simulink model "Karnop"  (R2015b)
settings: Solver=VariableStepAuto  StartTime=0.0  StopTime=10.0  RelTol=1e-3
values from neighbouring files (symbols this model uses):
  d_v = 10    [ex1.m]    (also in ex2.m = 1; ex3.m; ex4.m = 1; exall.m = 1)
  F_c = 0.001    [ex1.m]    (also in ex2.m; ex3.m; ex4.m; exall.m)
  motor_L = motor_pars    [ex1.m]    (also in ex2.m; ex3.m; ex4.m)
libraries: simulink x1
settings Model: Creator=Andreas  LastModifiedBy=Andreas

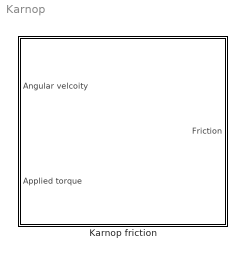
== system Karnop ==
  Karnop friction : Subsystem

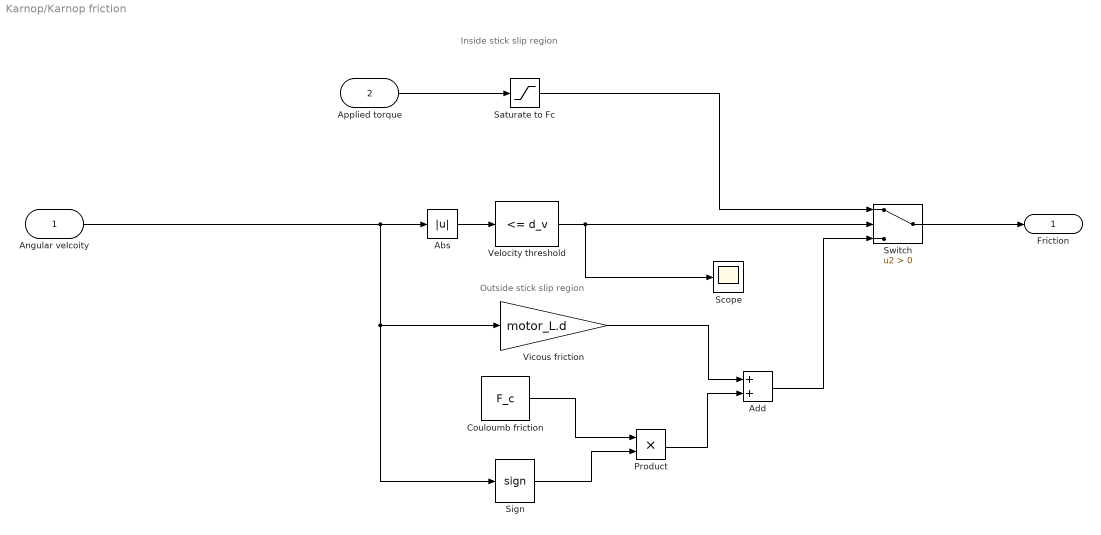
== system Karnop/Karnop friction ==
  note: Outside stick slip region
  note: Inside stick slip region
  Angular velcoity : Inport
  "Applied torque " : Inport  Port=2
  Abs : Abs
  Add : Sum
  Couloumb friction : Constant  Value=F_c
  Product : Product
  Saturate to Fc : Saturate  UpperLimit=F_c  LowerLimit=-F_c
  Scope : Scope
  Sign : Signum
  Switch : Switch  Criteria=u2 > Threshold
  "Velocity threshold " : simulink/Logic and Bit Operations/Compare To Constant  relop=<=  const=d_v  OutDataTypeStr=uint8
  Vicous friction : Gain  Gain=motor_L.d
  Friction : Outport
  wires:
  Add/1 -> Switch/3
  "Applied torque "/1 -> Saturate to Fc/1
  Sign/1 -> Product/2
  Couloumb friction/1 -> Product/1
  Vicous friction/1 -> Add/1
  Product/1 -> Add/2
  Abs/1 -> "Velocity threshold "/1
  "Velocity threshold "/1 -> Switch/2, Scope/1
  Angular velcoity/1 -> Sign/1, Vicous friction/1, Abs/1
  Switch/1 -> Friction/1
  Saturate to Fc/1 -> Switch/1
